simulink model "heating_cooling_control"  (Simulink 3.00)
libraries: mathlib x6, arclib x3, genlib x2, reglib x2

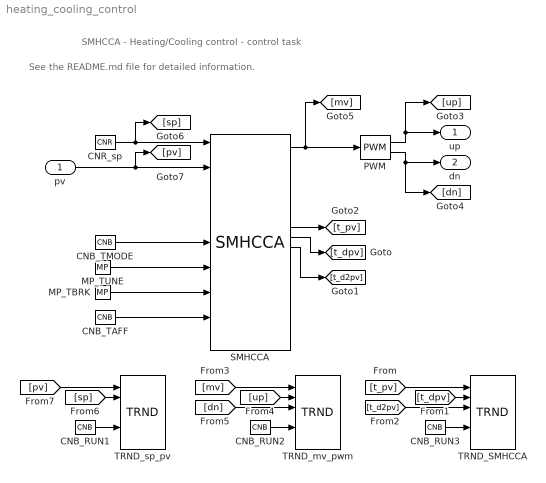
== system heating_cooling_control ==
  note: See the README.md file for detailed information.
  note: SMHCCA - Heating/Cooling control - control task
  pv : Inport  Port=1
  CNB_RUN1 : mathlib/CNB  YCN=on
  CNB_RUN2 : mathlib/CNB  YCN=on
  CNB_RUN3 : mathlib/CNB  YCN=on
  CNB_TAFF : mathlib/CNB  YCN=on
  CNB_TMODE : mathlib/CNB  YCN=on
  CNR_sp : mathlib/CNR  ycn=300
  MP_TBRK : genlib/MP  pwidth=1  BSTATE=off  RPTF=off
  MP_TUNE : genlib/MP  pwidth=1  BSTATE=on  RPTF=off
  PWM : reglib/PWM  pertm=1  dtime=0.01  btime=0.01  offtime=0.01  asyfac=1  SYNCH=off
  SMHCCA : reglib/SMHCCA  ipwmc=100  xi=1  om=0.01  taup=50  taum=30  beta=0.01  hilim_p=1  hilim_m=1  u0_p=1  u0_m=1  sp_dif=10  tauf=30  itm=1: Restricted to symmetrical processes  ut_p=1  ut_m=1
  TRND_SMHCCA : arclib/TRND  n=3  l=100000  btype=8: Double  ptype1=1: Store  ptype2=1: Store  ptype3=1: Store  ptype4=1: Store  pfac=1  afac=0  arc=0  id=1  Title=Trend Title  timesrc=1
  TRND_mv_pwm : arclib/TRND  n=3  l=100000  btype=8: Double  ptype1=1: Store  ptype2=1: Store  ptype3=1: Store  ptype4=1: Store  pfac=1  afac=0  arc=0  id=1  Title=Trend Title  timesrc=1
  TRND_sp_pv : arclib/TRND  n=2  l=100000  btype=8: Double  ptype1=1: Store  ptype2=1: Store  ptype3=1: Store  ptype4=1: Store  pfac=1  afac=0  arc=0  id=1  Title=Trend Title  timesrc=1
  up : Outport  Port=1
  dn : Outport  Port=2
  wires:
  CNB_RUN1/1 -> TRND_sp_pv/5
  CNB_RUN2/1 -> TRND_mv_pwm/5
  CNB_RUN3/1 -> TRND_SMHCCA/5
  CNB_TAFF/1 -> SMHCCA/8
  CNB_TMODE/1 -> SMHCCA/5
  CNR_sp/1 -> [sp], SMHCCA/1
  [t_pv] -> TRND_SMHCCA/1
  [t_dpv] -> TRND_SMHCCA/2
  [t_d2pv] -> TRND_SMHCCA/3
  [mv] -> TRND_mv_pwm/1
  [up] -> TRND_mv_pwm/2
  [dn] -> TRND_mv_pwm/3
  [sp] -> TRND_sp_pv/2
  [pv] -> TRND_sp_pv/1
  MP_TBRK/1 -> SMHCCA/7
  MP_TUNE/1 -> SMHCCA/6
  PWM/1 -> [up], up/1
  PWM/2 -> [dn], dn/1
  SMHCCA/1 -> [mv], PWM/1
  SMHCCA/9 -> [t_pv]
  SMHCCA/10 -> [t_dpv]
  SMHCCA/11 -> [t_d2pv]
  pv/1 -> [pv], SMHCCA/2
